simulink model "DFC4PIDLab2019b"  (R2019b)
settings: Solver=VariableStepAuto  StartTime=0.0  StopTime=inf  RelTol=1e-3
undefined symbols (not defined in the file or in its folder): daq
libraries: daqlib x2
settings Model: Creator=875549  LastModifiedBy=onura

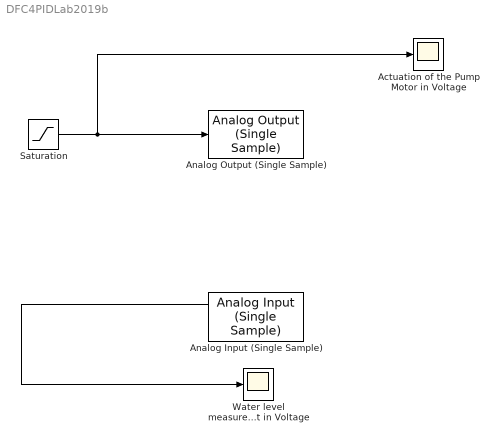
== system DFC4PIDLab2019b ==
  Actuation of the Pump Motor in Voltage : Scope
  Analog Input (Single Sample) : daqlib/Analog Input (Single Sample)  DeviceMenu=(none)  Device=ni myDAQ1 (NI myDAQ)  ObjConstructor=daq.createSession('ni')  BlockSampleTime=0.01  NChannelsSelected=1  Channels=1$ai0$$myDAQ1$1$2$1$1$#0$ai1$$myDAQ1$1$2$1$1$#  NPorts=1 for all channels  OutputTimestamp=on
      settings: SourceProductBaseCode=DA
  Analog Output (Single Sample) : daqlib/Analog Output (Single Sample)  DeviceMenu=(none)  Device=ni myDAQ1 (NI myDAQ)  ObjConstructor=daq.createSession('ni')  NChannelsSelected=1  Channels=1$ao0$$myDAQ1$1$2$N/A$#0$ao1$$myDAQ1$1$2$N/A$#  NPorts=1 for all channels  BlockSampleTime=.01
      settings: SourceProductBaseCode=DA
  Saturation : Saturate  UpperLimit=10  LowerLimit=-10
  Water level measurement in Voltage : Scope
  wires:
  Analog Input (Single Sample)/1 -> Water level measurement in Voltage/1
  Saturation/1 -> Analog Output (Single Sample)/1, Actuation of the Pump Motor in Voltage/1
